simulink model "RngMod_TrqSpdCrv"  (R2016b)
settings: configuration reference "CodeGenConfigSet" (kept outside this file)
values from neighbouring files (symbols this model uses):
  RngMod_trqCrSMax_CUR = Calibration.Parameter    [init_RngMod_TrqSpdCrv.m]
  RngMod_trqCrSMax_CURX = Calibration.Parameter    [init_RngMod_TrqSpdCrv.m]
  RngMod_trqMax_CUR = Calibration.Parameter    [init_RngMod_TrqSpdCrv.m]
  RngMod_trqMax_CURX = Calibration.Parameter    [init_RngMod_TrqSpdCrv.m]
undefined symbols (not defined in the file or in its folder): HPUn_etaPmp_MAPY
settings Model: Creator=Wollf  LastModifiedBy=wangrui
settings ConfigSetRef: SourceLocation=Base Workspace

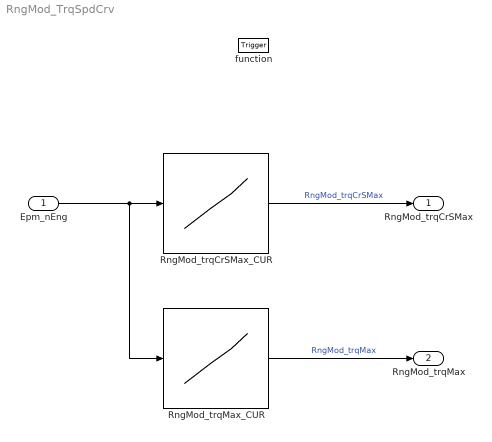
== system RngMod_TrqSpdCrv ==
  Epm_nEng : Inport  Tag=rpm  Description=Engine speed  OutMin=0  OutMax=6000  OutDataTypeStr=EngSpeed_rpm
  function : TriggerPort  TriggerType=function-call  VariantControl=Variant
  RngMod_trqCrSMax_CUR : Lookup_n-D  NumberOfTableDimensions=1  BreakpointsForDimension1=RngMod_trqCrSMax_CURX  BreakpointsForDimension2=HPUn_etaPmp_MAPY  IndexSearchMethod=Linear search  BeginIndexSearchUsingPreviousIndexResult=on  Table=RngMod_trqCrSMax_CUR  ExtrapMethod=Clip  UseLastTableValue=on  InternalRulePriority=Speed  OutDataTypeStr=Inherit: Inherit via back propagation  SaturateOnIntegerOverflow=on
  RngMod_trqMax_CUR : Lookup_n-D  NumberOfTableDimensions=1  BreakpointsForDimension1=RngMod_trqMax_CURX  BreakpointsForDimension2=HPUn_etaPmp_MAPY  IndexSearchMethod=Linear search  BeginIndexSearchUsingPreviousIndexResult=on  Table=RngMod_trqMax_CUR  ExtrapMethod=Clip  UseLastTableValue=on  InternalRulePriority=Speed  OutDataTypeStr=Inherit: Inherit via back propagation  SaturateOnIntegerOverflow=on
  RngMod_trqCrSMax : Outport  Tag=Nm  Description=maximal crankshaft torque  OutMin=-3276.8  OutMax=3276.7  OutDataTypeStr=Trq_Nm
  RngMod_trqMax : Outport  Tag=Nm  Description=Maximum of torque interval  Port=2  OutMin=-3276.8  OutMax=3276.7  OutDataTypeStr=Trq_Nm
  wires:
  Epm_nEng/1 -> RngMod_trqMax_CUR/1, RngMod_trqCrSMax_CUR/1
  RngMod_trqCrSMax_CUR/1 -> RngMod_trqCrSMax/1  "RngMod_trqCrSMax"
  RngMod_trqMax_CUR/1 -> RngMod_trqMax/1  "RngMod_trqMax"
